simulink model "buck_simulation_1"  (R2023a)
settings: Solver=FixedStepAuto  StartTime=0.0  StopTime=0.5  FixedStep=1e-8  MaxStep=10e-9  RelTol=4e-3
libraries: spsSeriesRLCBranchLib x7, dspstat3 x6, spsDCVoltageSourceLib x2, spsMosfetLib x2, spsFourierLib x2, simulink x1, spsCurrentMeasurementLib x1, spsVoltageMeasurementLib x1, sps_lib x1
settings Model: Creator=13520  LastModifiedBy=13520

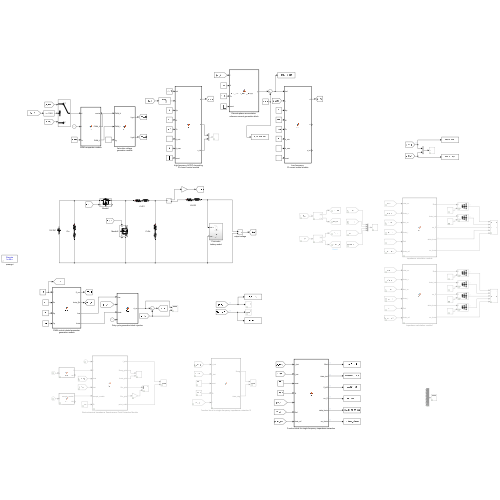
[thumbnail: Simulink's stored preview of the top-level diagram]
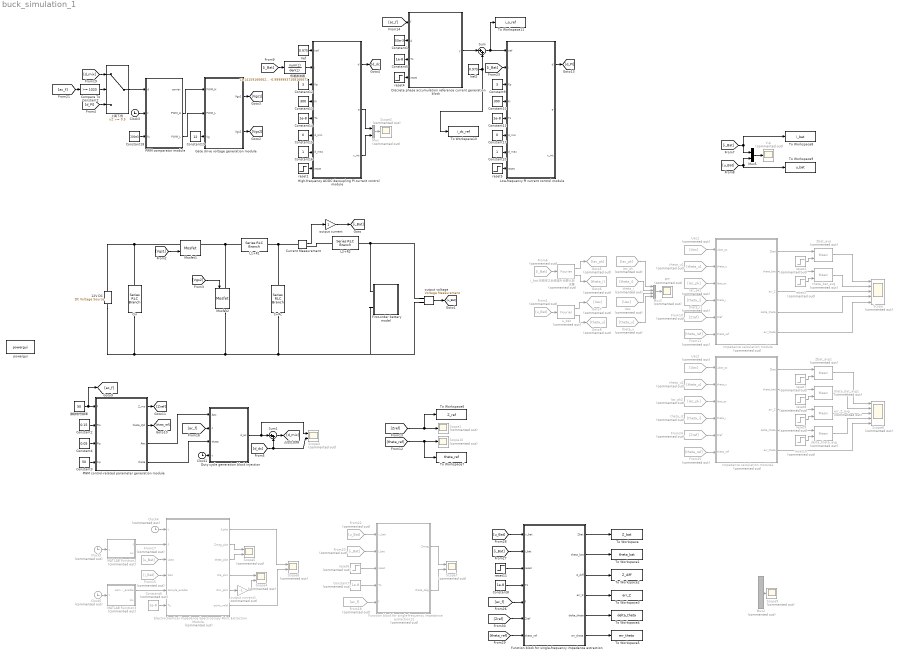
== system buck_simulation_1 ==
  12V DC : spsDCVoltageSourceLib/DC Voltage Source  Amplitude=12  Measurements=None
  C+Rc : spsSeriesRLCBranchLib/Series RLC Branch  LConnTagsString=__new0  RConnTagsString=__new0  BranchType=RC  Resistance=5e-1  Inductance=1e-3  SetiL0=off  InitialCurrent=0  Capacitance=220e-6  Setx0=off  InitialVoltage=0  Measurements=None
  Cin : spsSeriesRLCBranchLib/Series RLC Branch  LConnTagsString=__new0  RConnTagsString=__new0  BranchType=RC  Resistance=1  Inductance=1e-3  SetiL0=off  InitialCurrent=0  Capacitance=21e-6  Setx0=off  InitialVoltage=0  Measurements=None
  Clock1 : Clock
  Clock2 : Clock  Commented=on
  Clock3 : Clock
  Clock4 : Clock  Commented=on
  Clock5 : Clock  Commented=on
  Compare To Constant2 : simulink/Logic and Bit Operations/Compare To Constant  relop=>=  const=1020  OutDataTypeStr=boolean
  Constant1 : Constant  Value=50e-3
  Constant10 : Constant  Value=300
  Constant{5,8,11,14} (4 alike) : Constant  Value=1e-8
  Constant12 : Constant  Value=3
  Constant13 : Constant  Value=300
  Constant15 : Constant  Value=0
  Constant16 : Constant
  Constant17 : Constant  Value=0
  Constant18 : Constant  Value=200e3
  Constant19 : Constant  Value=12
  Constant2 : Constant  Value=0.15
  Constant20 : Constant
  Constant3 : Constant  Value=50
  Constant4 : Constant  Value=0.05
  Constant6 : Constant  Commented=on  Value=1e-8
  Constant7 : Constant  Commented=on  Value=1e-8
  Constant9 : Constant  Value=3
  Current Measurement : spsCurrentMeasurementLib/Current Measurement  PhasorSimulation=off  OutputType=Complex  PSBequivalent=0
  Discrete phase accumulation reference current generation block : MATLAB Function  TreatAsAtomicUnit=on
  Duty cycle generation block injection : MATLAB Function  TreatAsAtomicUnit=on
  Electrochemical Impedance Spectroscopy Point Extraction Module : MATLAB Function  Commented=on  TreatAsAtomicUnit=on
  FFT : Scope  Commented=on
  First-order battery model : Subsystem
  From1 : From  Commented=on  GotoTag=u_Bat
  From10 : From  Commented=on  GotoTag=Zref
  From11 : From  Commented=on  GotoTag=theta_ref
  From15 : From  Commented=on  GotoTag=i_Bat
  From17 : From  Commented=on  GotoTag=u_Bat
  From18 : From  Commented=on  GotoTag=ac_f
  From20 : From  Commented=on  GotoTag=i_Bat
  From22 : From  Commented=on  GotoTag=u_Bat
  From24 : From  Commented=on  GotoTag=Zref
  From25 : From  Commented=on  GotoTag=theta_ref
  From6 : From  Commented=on  GotoTag=i_Bat
  Function block for single-frequency impedance extraction : MATLAB Function  TreatAsAtomicUnit=on
  Function block for single-frequency impedance extraction12 : MATLAB Function  Commented=on  TreatAsAtomicUnit=on
  Gate drive voltage generation module : MATLAB Function  TreatAsAtomicUnit=on
  Goto5 : Goto  Commented=on  GotoTag=Iac_pk
  Goto6 : Goto  Commented=on  GotoTag=theta_i
  Goto7 : Goto  Commented=on  GotoTag=Uac
  Goto8 : Goto  Commented=on  GotoTag=theta_u
  High-frequency AC/DC decoupling PI current control module : MATLAB Function  TreatAsAtomicUnit=on  SystemSampleTime=1e-8
  Iac_pk : From  Commented=on  GotoTag=Iac_pk
  Iac_pk1 : From  Commented=on  GotoTag=Iac_pk
  Iac_pk2 : From  Commented=on  GotoTag=Iac_pk
  Impedance calculation module : MATLAB Function  Commented=on  TreatAsAtomicUnit=on
  Impedance calculation module1 : MATLAB Function  Commented=on  TreatAsAtomicUnit=on
  Iref : Constant  Value=0.975
  Iref2 : Constant  Value=0.975
  L1+R1 : spsSeriesRLCBranchLib/Series RLC Branch  LConnTagsString=__new0  RConnTagsString=__new0  BranchType=RL  Resistance=1e-1  Inductance=100e-6  SetiL0=off  InitialCurrent=0  Capacitance=1e-6  Setx0=off  InitialVoltage=0  Measurements=None
  L2+R2 : spsSeriesRLCBranchLib/Series RLC Branch  LConnTagsString=__new0  RConnTagsString=__new0  BranchType=RL  Resistance=16e-3  Inductance=15e-6  SetiL0=off  InitialCurrent=0  Capacitance=1e-6  Setx0=off  InitialVoltage=0  Measurements=None
  Low-frequency PI current control module : MATLAB Function  TreatAsAtomicUnit=on  SystemSampleTime=1e-8
  MATLAB Function2 : MATLAB Function  Commented=on  TreatAsAtomicUnit=on
  MATLAB Function3 : MATLAB Function  Commented=on  TreatAsAtomicUnit=on
  Mosfet1 : spsMosfetLib/Mosfet  Ron=0.1  Lon=0  Rd=0.01  Vfd=0  IC=0  Rs=1e5  Cs=inf  Measurements=on
  Mosfet2 : spsMosfetLib/Mosfet  Ron=0.1  Lon=0  Rd=0.01  Vfd=0  IC=0  Rs=1e5  Cs=inf  Measurements=on
  Mux : Mux  Commented=on  Inputs=2
  Mux1 : Mux  Commented=on
  Mux2 : Mux  Commented=on  Inputs=6
  Mux5 : Mux  Inputs=2
  PWM comparator module : MATLAB Function  TreatAsAtomicUnit=on
  PWM control-related parameter generation module : MATLAB Function  TreatAsAtomicUnit=on
  Scope : Scope  Commented=on  NumInputPorts=5
  Scope{1..2,9..10} (4 alike) : Scope  Commented=on
  Scope{3..7} (5 alike) : Scope  Commented=on  NumInputPorts=2
  Scope8 : Scope  Commented=on  NumInputPorts=5
  Sum : Sum  Inputs=|++
  Sum1 : Sum  Inputs=|++
  To Workspace : ToWorkspace  VariableName=Z_bat  SaveFormat=Timeseries  SampleTime=-1
  To Workspace1 : ToWorkspace  VariableName=theta_bat  SaveFormat=Timeseries  SampleTime=-1
  To Workspace10 : ToWorkspace  VariableName=i_dc_ref  SaveFormat=Timeseries  SampleTime=-1
  To Workspace11 : ToWorkspace  VariableName=i_o_ref  SaveFormat=Timeseries  SampleTime=-1
  To Workspace2 : ToWorkspace  VariableName=Z_diff  SaveFormat=Timeseries  SampleTime=-1
  To Workspace3 : ToWorkspace  VariableName=err_Z  SaveFormat=Timeseries  SampleTime=-1
  To Workspace4 : ToWorkspace  VariableName=delta_theta  SaveFormat=Timeseries  SampleTime=-1
  To Workspace5 : ToWorkspace  VariableName=err_theta  SaveFormat=Timeseries  SampleTime=-1
  To Workspace6 : ToWorkspace  VariableName=Z_ref  SaveFormat=Timeseries  SampleTime=-1
  To Workspace7 : ToWorkspace  VariableName=theta_ref  SaveFormat=Timeseries  SampleTime=-1
  To Workspace8 : ToWorkspace  VariableName=i_bat  SaveFormat=Timeseries  SampleTime=-1
  To Workspace9 : ToWorkspace  VariableName=u_bat  SaveFormat=Timeseries  SampleTime=-1
  Uac : From  Commented=on  GotoTag=Uac
  Uac1 : From  Commented=on  GotoTag=Uac
  Uac2 : From  Commented=on  GotoTag=Uac
  V-A : Scope  Commented=on
  Zbat_avg : dspstat3/Mean  Commented=on  run=on  reset_popup=Rising edge  directionMode=Each column  dimension=1  roiEnable=off  roiType=Rectangles  roiPortion=Entire ROI  roiOutput=Individual statistics for each ROI  roiFlag=off  roundingMode=Floor  overflowMode=off  outputDataTypeStr=Inherit: Same as accumulator  outputMin=[]  outputMax=[]  outputLastDataTypeStr=Inherit: Same as accumulator
  Zbat_avg1 : dspstat3/Mean  Commented=on  run=on  reset_popup=Rising edge  directionMode=Each column  dimension=1  roiEnable=off  roiType=Rectangles  roiPortion=Entire ROI  roiOutput=Individual statistics for each ROI  roiFlag=off  roundingMode=Floor  overflowMode=off  outputDataTypeStr=Inherit: Same as accumulator  outputMin=[]  outputMax=[]  outputLastDataTypeStr=Inherit: Same as accumulator
  delta_theta_avg : dspstat3/Mean  Commented=on  run=on  reset_popup=Rising edge  directionMode=Each column  dimension=1  roiEnable=off  roiType=Rectangles  roiPortion=Entire ROI  roiOutput=Individual statistics for each ROI  roiFlag=off  roundingMode=Floor  overflowMode=off  outputDataTypeStr=Inherit: Same as accumulator  outputMin=[]  outputMax=[]  outputLastDataTypeStr=Inherit: Same as accumulator
  err_Z_avg : dspstat3/Mean  Commented=on  run=on  reset_popup=Rising edge  directionMode=Each column  dimension=1  roiEnable=off  roiType=Rectangles  roiPortion=Entire ROI  roiOutput=Individual statistics for each ROI  roiFlag=off  roundingMode=Floor  overflowMode=off  outputDataTypeStr=Inherit: Same as accumulator  outputMin=[]  outputMax=[]  outputLastDataTypeStr=Inherit: Same as accumulator
  i_bat 改频率之后傅里叶也要从新设置 : spsFourierLib/Fourier  Commented=on  Freq=50  n=1  InInit=[0, 0]  Ts=1e-8
  output current : Gain
  output current1 : Gain  Commented=on  Gain=-1
  output voltage : spsVoltageMeasurementLib/Voltage Measurement  PhasorSimulation=off  OutputType=Complex  PSBequivalent=0
  powergui : sps_lib/powergui  Priority=1  SimulationMode=Discrete  SampleTime=1e-8  frequency=60  Iterations=50  frequencyindice=0  Pbase=100e6  ErrMax=1e-4  UnitsV=kV  UnitsW=MW  buscounter=0  FunctionMessages=off  echomessages=off  EnableUseOfTLC=off  CurrentSourceSwitches=off  DisableSnubberDevices=off  DisableRonSwitches=off  DisableVfSwitches=off  DisplayEquations=off  AutomaticDiscreteSolvers=off  SolverType=Tustin/Backward Euler (TBE)  Interpol=off  ExternalGateDelay=off  methode=off  Ts=100  x0status=blocks  SPID=on  SwTol=0  HookPort=off  NonlinearTolerance=1e-4  nMaxIteration=100  ContinueOnMaxIteration=off  RestoreLinks=warning  ResistiveCurrentMeasurement=off  Frange=[0:2:500]  Ylog=off  Xlog=on  ShowGrid=off  save=off  variable=ZData  structure=0  ZoomFFT=off  StartTime=0.0  cycles=1  DisplayStyle=1  fundamental=60  FreqAxis=off  MaxFrequency=1000  frequencyindicesteady=1  RmsSteady=1  display=off
  reset1 : Step  Time=0  Before=1  After=0  SampleTime=0
  reset{7..10} (4 alike) : Step  Commented=on  Time=0.05  SampleTime=1e-8
  reset11 : Step  Time=0.1  Before=1  After=0  SampleTime=0
  reset2 : Step  Commented=on  Time=0.25  SampleTime=1e-8
  reset3 : Step  Commented=on  Time=0.25  SampleTime=1e-8
  reset4 : Step  Time=0.05  Before=1  After=0  SampleTime=0
  reset5 : Step  Time=0  Before=1  After=0  SampleTime=0
  reset6 : Step  Commented=on  Time=0.1  Before=1  After=0  SampleTime=0
  theta_bat_avg : dspstat3/Mean  Commented=on  run=on  reset_popup=Rising edge  directionMode=Each column  dimension=1  roiEnable=off  roiType=Rectangles  roiPortion=Entire ROI  roiOutput=Individual statistics for each ROI  roiFlag=off  roundingMode=Floor  overflowMode=off  outputDataTypeStr=Inherit: Same as accumulator  outputMin=[]  outputMax=[]  outputLastDataTypeStr=Inherit: Same as accumulator
  theta_bat_avg1 : dspstat3/Mean  Commented=on  run=on  reset_popup=Rising edge  directionMode=Each column  dimension=1  roiEnable=off  roiType=Rectangles  roiPortion=Entire ROI  roiOutput=Individual statistics for each ROI  roiFlag=off  roundingMode=Floor  overflowMode=off  outputDataTypeStr=Inherit: Same as accumulator  outputMin=[]  outputMax=[]  outputLastDataTypeStr=Inherit: Same as accumulator
  theta_i : From  Commented=on  GotoTag=theta_i
  theta_i1 : From  Commented=on  GotoTag=theta_i
  theta_i2 : From  Commented=on  GotoTag=theta_i
  theta_u : From  Commented=on  GotoTag=theta_u
  theta_u1 : From  Commented=on  GotoTag=theta_u
  theta_u2 : From  Commented=on  GotoTag=theta_u
  u_bat : spsFourierLib/Fourier  Commented=on  Freq=50  n=1  InInit=[0, 0]  Ts=1e-8
  上高下低 : Switch  Threshold=0.5  SaturateOnIntegerOverflow=off  InputSameDT=off
  低通滤波器 : DiscreteTransferFcn  Numerator=[3.141591666629663e-07 3.141591666629663e-07]  Denominator=[1 -0.9999993716816667]  SampleTime=1e-8
  激励信号频率 : Constant  Value=50
  wires:
  Mux/1 -> Scope2/1
  [Vgs1] -> Mosfet1/1
  Constant12/1 -> High-frequency AC/DC decoupling PI current control module/3(Kp)
  Constant13/1 -> High-frequency AC/DC decoupling PI current control module/4(Ki)
  Constant14/1 -> High-frequency AC/DC decoupling PI current control module/5(Ts)
  Constant15/1 -> High-frequency AC/DC decoupling PI current control module/6(d_min)
  Constant16/1 -> High-frequency AC/DC decoupling PI current control module/7(d_max)
  reset1/1 -> High-frequency AC/DC decoupling PI current control module/8(reset)
  Constant19/1 -> Gate drive voltage generation module/3(Vg)
  PWM comparator module/2(PWM_H) -> Gate drive voltage generation module/1(PWM_H)
  PWM comparator module/3(PWM_L) -> Gate drive voltage generation module/2(PWM_L)
  Clock3/1 -> PWM comparator module/2(t)
  Constant18/1 -> PWM comparator module/3(fs)
  Gate drive voltage generation module/2(Vgs2) -> [Vgs2]
  Gate drive voltage generation module/1(Vgs1) -> [Vgs1]
  [Vgs2] -> Mosfet2/1
  Mux5/1 -> V-A/1
  output voltage/1 -> [u_Bat]
  Current Measurement/1 -> output current/1
  output current/1 -> [i_Bat]
  High-frequency AC/DC decoupling PI current control module/2(e) -> Mux/1
  High-frequency AC/DC decoupling PI current control module/3(x_int) -> Mux/2
  From1/1 -> u_bat/1
  From6/1 -> i_bat 改频率之后傅里叶也要从新设置/1
  [i_Bat] -> Mux5/1, To Workspace8/1
  [u_Bat] -> Mux5/2, To Workspace9/1
  i_bat 改频率之后傅里叶也要从新设置/1 -> Goto5/1
  i_bat 改频率之后傅里叶也要从新设置/2 -> Goto6/1
  u_bat/1 -> Goto7/1
  u_bat/2 -> Goto8/1
  Mux1/1 -> FFT/1
  Iac_pk/1 -> Mux1/1
  theta_i/1 -> Mux1/2
  Uac/1 -> Mux1/3
  theta_u/1 -> Mux1/4
  Uac1/1 -> Impedance calculation module/1(ubat_ac)
  Iac_pk1/1 -> Impedance calculation module/3(ibat_ac)
  theta_u1/1 -> Impedance calculation module/2(theta_u)
  theta_i1/1 -> Impedance calculation module/4(theta_i)
  From10/1 -> Impedance calculation module/5(Zref)
  Constant2/1 -> PWM control-related parameter generation module/2(Ro)
  Constant4/1 -> PWM control-related parameter generation module/3(Rp)
  Constant3/1 -> PWM control-related parameter generation module/4(Cp)
  PWM control-related parameter generation module/1(Z_mo) -> [Zref]
  From11/1 -> Impedance calculation module/6(theta_ref)
  PWM control-related parameter generation module/2(theta_Zjd) -> [theta_ref]
  [Zref] -> To Workspace6/1, Scope1/1
  [theta_ref] -> To Workspace7/1, Scope10/1
  reset2/1 -> Zbat_avg/2
  Impedance calculation module/1(Zbat) -> Zbat_avg/1
  reset3/1 -> theta_bat_avg/2
  Impedance calculation module/2(theta_bat) -> theta_bat_avg/1
  Zbat_avg/1 -> Scope/1
  theta_bat_avg/1 -> Scope/2
  Impedance calculation module/3(err_Z) -> Scope/3
  Impedance calculation module/4(delta_theta) -> Scope/4
  Impedance calculation module/5(err_theta) -> Scope/5
  [i_Bat] -> 低通滤波器/1
  Clock1/1 -> Duty cycle generation block injection/4(t)
  Iref/1 -> High-frequency AC/DC decoupling PI current control module/1(Iref)
  低通滤波器/1 -> High-frequency AC/DC decoupling PI current control module/2(i)
  PWM control-related parameter generation module/3(Aac) -> Duty cycle generation block injection/1(Aac)
  PWM control-related parameter generation module/4(theta) -> Duty cycle generation block injection/3(theta)
  [d_dc] -> Sum1/2, Scope3/2
  Sum1/1 -> [d_mix]
  Duty cycle generation block injection/1(d_ac) -> Scope3/1, Sum1/1
  High-frequency AC/DC decoupling PI current control module/1(d) -> [d_dc]
  Compare To Constant2/1 -> 上高下低/2
  上高下低/1 -> PWM comparator module/1(d)
  [ac_f] -> Compare To Constant2/1
  Constant11/1 -> Low-frequency PI current control module/5(Ts)
  Constant9/1 -> Low-frequency PI current control module/3(Kp)
  Constant17/1 -> Low-frequency PI current control module/6(d_min)
  Constant10/1 -> Low-frequency PI current control module/4(Ki)
  reset5/1 -> Low-frequency PI current control module/8(reset)
  Constant20/1 -> Low-frequency PI current control module/7(d_max)
  [ac_f] -> Duty cycle generation block injection/2(f)
  Low-frequency PI current control module/1(d) -> [d_PI]
  [d_mix] -> 上高下低/1
  [d_PI] -> 上高下低/3
  [i_Bat] -> Low-frequency PI current control module/2(i)
  Sum/1 -> To Workspace11/1, Low-frequency PI current control module/1(Iref)
  Iref2/1 -> Sum/2, To Workspace10/1
  Discrete phase accumulation reference current generation block/1(y) -> Sum/1
  [ac_f] -> Discrete phase accumulation reference current generation block/1(f)
  Constant1/1 -> Discrete phase accumulation reference current generation block/2(A)
  Constant5/1 -> Discrete phase accumulation reference current generation block/3(Ts)
  reset4/1 -> Discrete phase accumulation reference current generation block/4(reset)
  MATLAB Function3/1(sample_enable) -> Electrochemical Impedance Spectroscopy Point Extraction Module/5(sample_enable)
  Clock2/1 -> MATLAB Function2/1(t)
  Clock4/1 -> Electrochemical Impedance Spectroscopy Point Extraction Module/1(t)
  Clock5/1 -> MATLAB Function3/1(t)
  From17/1 -> Electrochemical Impedance Spectroscopy Point Extraction Module/3(ubat)
  From15/1 -> Electrochemical Impedance Spectroscopy Point Extraction Module/4(ibat)
  Constant6/1 -> Electrochemical Impedance Spectroscopy Point Extraction Module/6(Ts)
  Electrochemical Impedance Spectroscopy Point Extraction Module/4(Zre_plot) -> Scope4/1
  Electrochemical Impedance Spectroscopy Point Extraction Module/5(Zim_plot) -> output current1/1
  output current1/1 -> Scope4/2
  Electrochemical Impedance Spectroscopy Point Extraction Module/2(Zmag_plot) -> Scope5/1
  Electrochemical Impedance Spectroscopy Point Extraction Module/3(theta_plot) -> Scope5/2
  Electrochemical Impedance Spectroscopy Point Extraction Module/1(f_plot) -> Scope6/1
  Electrochemical Impedance Spectroscopy Point Extraction Module/6(point_valid) -> Scope6/2
  MATLAB Function2/1(f) -> Electrochemical Impedance Spectroscopy Point Extraction Module/2(f)
  激励信号频率/1 -> [ac_f], PWM control-related parameter generation module/1(f)
  From18/1 -> Function block for single-frequency impedance extraction12/5(f)
  Constant7/1 -> Function block for single-frequency impedance extraction12/4(Ts)
  From22/1 -> Function block for single-frequency impedance extraction12/1(v_bat)
  From20/1 -> Function block for single-frequency impedance extraction12/2(i_bat)
  reset6/1 -> Function block for single-frequency impedance extraction12/3(reset)
  Function block for single-frequency impedance extraction12/1(Zmag) -> Scope7/1
  Function block for single-frequency impedance extraction12/2(theta_deg) -> Scope7/2
  theta_bat_avg1/1 -> Scope8/2
  reset8/1 -> theta_bat_avg1/2
  Impedance calculation module1/2(theta_bat) -> theta_bat_avg1/1
  Impedance calculation module1/5(err_theta) -> Scope8/5
  Zbat_avg1/1 -> Scope8/1
  Impedance calculation module1/1(Zbat) -> Zbat_avg1/1
  Iac_pk2/1 -> Impedance calculation module1/3(ibat_ac)
  From24/1 -> Impedance calculation module1/5(Zref)
  From25/1 -> Impedance calculation module1/6(theta_ref)
  theta_u2/1 -> Impedance calculation module1/2(theta_u)
  theta_i2/1 -> Impedance calculation module1/4(theta_i)
  reset7/1 -> Zbat_avg1/2
  Uac2/1 -> Impedance calculation module1/1(ubat_ac)
  reset9/1 -> err_Z_avg/2
  Impedance calculation module1/3(err_Z) -> err_Z_avg/1
  err_Z_avg/1 -> Scope8/3
  reset10/1 -> delta_theta_avg/2
  Impedance calculation module1/4(delta_theta) -> delta_theta_avg/1
  delta_theta_avg/1 -> Scope8/4
  Constant8/1 -> Function block for single-frequency impedance extraction/4(Ts)
  reset11/1 -> Function block for single-frequency impedance extraction/3(reset)
  [u_Bat] -> Function block for single-frequency impedance extraction/1(v_bat)
  [i_Bat] -> Function block for single-frequency impedance extraction/2(i_bat)
  [ac_f] -> Function block for single-frequency impedance extraction/5(f)
  Mux2/1 -> Scope9/1
  Function block for single-frequency impedance extraction/4(err_Z) -> To Workspace3/1
  Function block for single-frequency impedance extraction/2(theta_bat) -> To Workspace1/1
  Function block for single-frequency impedance extraction/1(Zbat) -> To Workspace/1
  Function block for single-frequency impedance extraction/5(delta_theta) -> To Workspace4/1
  Function block for single-frequency impedance extraction/6(err_theta) -> To Workspace5/1
  [Zref] -> Function block for single-frequency impedance extraction/6(Zref)
  [theta_ref] -> Function block for single-frequency impedance extraction/7(theta_ref)
  Function block for single-frequency impedance extraction/3(Z_diff) -> To Workspace2/1
  connections:
  12V DC/RConn1 -- Mosfet1/LConn1 -- Cin/LConn1
  L1+R1/LConn1 -- Mosfet2/LConn1 -- Mosfet1/RConn1
  C+Rc/LConn1 -- Current Measurement/LConn1 -- L1+R1/RConn1
  12V DC/LConn1 -- Cin/RConn1 -- Mosfet2/RConn1 -- output voltage/LConn2 -- First-order battery model/LConn2 -- C+Rc/RConn1
  L2+R2/LConn1 -- Current Measurement/RConn1
  output voltage/LConn1 -- First-order battery model/LConn1 -- L2+R2/RConn1

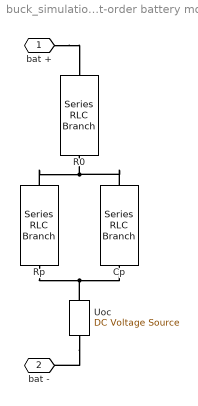
== system buck_simulation_1/First-order battery model ==
  Cp : spsSeriesRLCBranchLib/Series RLC Branch  LConnTagsString=__new0  RConnTagsString=__new0  BranchType=C  Resistance=0.5  Inductance=1e-3  SetiL0=off  InitialCurrent=0  Capacitance=50  Setx0=off  InitialVoltage=0  Measurements=None
  R0 : spsSeriesRLCBranchLib/Series RLC Branch  LConnTagsString=__new0  RConnTagsString=__new0  BranchType=R  Resistance=15e-2  Inductance=1e-3  SetiL0=off  InitialCurrent=0  Capacitance=1e-6  Setx0=off  InitialVoltage=0  Measurements=None
  Rp : spsSeriesRLCBranchLib/Series RLC Branch  LConnTagsString=__new0  RConnTagsString=__new0  BranchType=R  Resistance=5e-2  Inductance=1e-3  SetiL0=off  InitialCurrent=0  Capacitance=1e-6  Setx0=off  InitialVoltage=0  Measurements=None
  Uoc : spsDCVoltageSourceLib/DC Voltage Source  Amplitude=3.6  Measurements=None
  bat + : PMIOPort  Side=Left
  bat - : PMIOPort  Port=2  Side=Left
  connections:
  Rp/RConn1 -- Uoc/RConn1 -- Cp/RConn1
  Rp/LConn1 -- Cp/LConn1 -- R0/RConn1
  bat +/RConn1 -- R0/LConn1
  Uoc/LConn1 -- bat -/RConn1

== matlab function buck_simulation_1/High-frequency AC//DC decoupling PI current control module ==
  settings: updateMethod=DISCRETE
  data: Iref input; d output; i input; Kp input; Ki input; Ts input; d_min input; d_max input; reset input; e output; x_int output
function [d, e, x_int] = fcn(Iref, i, Kp, Ki, Ts, d_min, d_max, reset)
% High-frequency AC/DC decoupling PI current control module
% Inputs:
%   Iref  - Reference current
%   i     - Actual current
%   Kp    - Proportional coefficient
%   Ki    - Integral coefficient
%   Ts    - Sampling period
%   d_min - Lower duty cycle limit
%   d_max - Upper duty cycle limit
%   reset - Reset signal
%
% Outputs:
%   d     - Duty cycle output
%   e     - Current error
%   x_int - Integral state

persistent int_e

if isempty(int_e)
    int_e = 0;
end

if reset > 0.5
    int_e = 0;
end

% Current error
e = Iref - i;

% Integral term
int_e = int_e + e * Ts;

% PI output
d = Kp * e + Ki * int_e;

% Duty cycle saturation
if d > d_max
    d = d_max;
elseif d < d_min
    d = d_min;
end

% Output integral state
x_int = int_e;
end

== matlab function buck_simulation_1/Gate drive voltage generation module ==
  data: PWM_H input; Vgs1 output; PWM_L input; Vg input; Vgs2 output
function [Vgs1, Vgs2] = fcn(PWM_H, PWM_L, Vg)
% Gate drive voltage generation module
% Inputs:
%   PWM_H - High-side PWM (recommended input: 0 or 1)
%   PWM_L - Low-side PWM (recommended input: 0 or 1)
%   Vg    - Gate-source drive voltage amplitude, for example 12 V
%
% Outputs:
%   Vgs1  - Gate-source drive voltage of S1
%   Vgs2  - Gate-source drive voltage of S2

% Limit the high-side PWM to 0~1
if PWM_H >= 0.5
    h = 1;
else
    h = 0;
end

% Limit the low-side PWM to 0~1
if PWM_L >= 0.5
    l = 1;
else
    l = 0;
end

% Drive amplitude protection
if Vg < 0
    Vg_use = 0;
else
    Vg_use = Vg;
end

% Output gate-source voltage
Vgs1 = h * Vg_use;
Vgs2 = l * Vg_use;
end

== matlab function buck_simulation_1/MATLAB Function2 ==
  data: t input; f output; sw output
function [f, sw] = fcn(t)
% 扫频块 / 交流激励电流频率生成模块
% 输入:
%   t  - 当前仿真时间
%
% 输出:
%   f  - 当前扫频频率
%   sw - 附录1原始控制标志

% 附录1中的频率数组
fx = [1 25000 20000 10000 5000 2000 1000 500 50 10];

% 附录1中的时间切换点数组
tx = [0 0.1 0.69 1.09 1.64 2.29 3.24 4.69 6.09 8];

% 附录1中的控制标志数组
swx = [0 1 1 1 1 1 1 1 1 1];

% 默认输出最后一个频点
f = fx(10);
sw = swx(10);

for i = 1:length(tx)-1
    if t >= tx(i) && t <= tx(i+1)
        f = fx(i);
        sw = swx(i);
        break;
    end
end
end

== matlab function buck_simulation_1/MATLAB Function3 ==
  data: t input; sample_enable output; idx output
function [sample_enable, idx] = fcn(t)
% 扫频采样窗口生成模块
% 输入:
%   t - 当前仿真时间
%
% 输出:
%   sample_enable - 当前频点是否允许采样
%   idx           - 当前频点索引

% 附录1时间切换点
tx = [0 0.1 0.69 1.09 1.64 2.29 3.24 4.69 6.09 8];

sample_enable = 0;
idx = 0;

for i = 1:length(tx)-1
    if t >= tx(i) && t < tx(i+1)
        idx = i;
        t1 = tx(i);
        t2 = tx(i+1);

        % 只在该频点区间后20%允许采样
        if t >= t1 + 0.8*(t2 - t1)
            sample_enable = 1;
        end
        break;
    end
end
end

== matlab function buck_simulation_1/Function block for single-frequency impedance extraction12 ==
  data: v_bat input; Zmag output; i_bat input; reset input; Ts input; f input; theta_deg output
function [Zmag, theta_deg] = fcn(v_bat, i_bat, reset, Ts, f)
% 用于单频阻抗提的取函数块
% 输入:
%   v_bat   - 电池端电压
%   i_bat   - 电池端电流
%   reset   - 复位信号，1=清零并等待，0=开始测量
%   Ts      - 离散步长
%   f       - 当前激励频率(Hz)
%
% 输出:
%   Zmag      - 当前频点阻抗模
%   theta_deg - 当前频点阻抗角(度)
%
% 说明:
%   1) 该模块采用单频同步检波法，不需要额外 Fourier 块
%   2) reset=1 时清空内部状态，适合在 PI 稳定阶段保持复位
%   3) reset 拉低后，模块开始对当前频率进行多周期累计
%   4) 达到设定测量周期数后，输出并保持该频点结果

% ========= 可调参数 =========
N_cycle_measure = 3;    % 测量周期数，可改为 2~5
I_min = 1e-9;           % 防止除零
% ===========================

persistent phi
persistent t_acc
persistent vsum_sin vsum_cos isum_sin isum_cos
persistent sample_count
persistent Zmag_hold theta_hold

if isempty(phi)
    phi = 0;
    t_acc = 0;
    vsum_sin = 0;
    vsum_cos = 0;
    isum_sin = 0;
    isum_cos = 0;
    sample_count = 0;
    Zmag_hold = 0;
    theta_hold = 0;
end

% 默认输出保持上一次有效值
Zmag = Zmag_hold;
theta_deg = theta_hold;

% 频率非法时直接返回
if f <= 0 || Ts <= 0
    Zmag = 0;
    theta_deg = 0;
    return;
end

% 复位：清空累计器，但不输出测量结果
if reset > 0.5
    phi = 0;
    t_acc = 0;
    vsum_sin = 0;
    vsum_cos = 0;
    isum_sin = 0;
    isum_cos = 0;
    sample_count = 0;
    Zmag_hold = 0;
    theta_hold = 0;

    Zmag = 0;
    theta_deg = 0;
    return;
end

% 当前角频率
w = 2*pi*f;

% 相位累加
phi = phi + w*Ts;

% 相位限制到 0~2pi
if phi >= 2*pi
    phi = phi - 2*pi*floor(phi/(2*pi));
end

% 参考正弦/余弦
ref_sin = sin(phi);
ref_cos = cos(phi);

% 同步检波累计
vsum_sin = vsum_sin + v_bat * ref_sin;
vsum_cos = vsum_cos + v_bat * ref_cos;

isum_sin = isum_sin + i_bat * ref_sin;
isum_cos = isum_cos + i_bat * ref_cos;

sample_count = sample_count + 1;
t_acc = t_acc + Ts;

% 达到设定测量时长后计算一次结果
T_measure = N_cycle_measure / f;

if t_acc >= T_measure
    % 提取当前频率分量
    Vsin = 2 * vsum_sin / sample_count;
    Vcos = 2 * vsum_cos / sample_count;

    Isin = 2 * isum_sin / sample_count;
    Icos = 2 * isum_cos / sample_count;

    % 幅值
    Vamp = sqrt(Vsin*Vsin + Vcos*Vcos);
    Iamp = sqrt(Isin*Isin + Icos*Icos);

    % 相位
    theta_v = atan2(Vcos, Vsin);
    theta_i = atan2(Icos, Isin);

    % 阻抗计算
    if Iamp > I_min
        Zmag_hold = Vamp / Iamp;
        theta_hold = (theta_v - theta_i) * 180 / pi;
    else
        Zmag_hold = 0;
        theta_hold = 0;
    end

    % 相角限制到 -180 ~ 180 deg
    while theta_hold > 180
        theta_hold = theta_hold - 360;
    end
    while theta_hold < -180
        theta_hold = theta_hold + 360;
    end

    % 输出最新结果
    Zmag = Zmag_hold;
    theta_deg = theta_hold;

    % 计算完成后，重新开始累计下一轮
    % 如果你只想每次 reset 后测一次并保持，也可以把下面这段删掉
    phi = 0;
    t_acc = 0;
    vsum_sin = 0;
    vsum_cos = 0;
    isum_sin = 0;
    isum_cos = 0;
    sample_count = 0;
end
end

== matlab function buck_simulation_1/Impedance calculation module1 ==
  data: ubat_ac input; Zbat output; theta_u input; ibat_ac input; theta_i input; Zref input; theta_ref input; theta_bat output; err_Z output; delta_theta output; err_theta output
function [Zbat, theta_bat, err_Z, delta_theta, err_theta] = fcn(ubat_ac, theta_u, ibat_ac, theta_i, Zref, theta_ref)
% 阻抗计算模块（抑制 100 Hz 误差振荡优化版）
% 输入:
%   ubat_ac   - 锂电池两端交流响应电压幅值
%   theta_u   - 锂电池两端交流响应电压相位（度）
%   ibat_ac   - 锂电池输入交流电流幅值
%   theta_i   - 锂电池输入交流电流相位（度）
%   Zref      - 标准阻抗模
%   theta_ref - 标准阻抗角（度）
%
% 输出:
%   Zbat        - 实测阻抗模（平滑后）
%   theta_bat   - 实测阻抗角（平滑后，度）
%   err_Z       - 阻抗模误差百分比（平滑后）
%   delta_theta - 阻抗角绝对误差（平滑后，度）
%   err_theta   - 阻抗角误差百分比（平滑后）

% =========================
% 可调参数
% =========================
eps_I = 1e-12;          % 防止电流幅值过小
eps_Z = 1e-12;          % 防止参考阻抗过小
theta_ref_min = 1e-3;   % 参考相角过小时，不计算百分比误差

alpha_Z = 0.02;         % 阻抗模平滑系数，越小越稳，建议 0.01~0.05
alpha_th = 0.02;        % 阻抗角平滑系数，越小越稳，建议 0.01~0.05
beta_err = 0.02;        % 误差平滑系数，越小越稳，建议 0.01~0.05

% =========================
% 持久变量
% =========================
persistent is_init
persistent Z_filt
persistent th_cos_filt th_sin_filt
persistent eZ_filt eTh_filt

if isempty(is_init)
    is_init = 0;
    Z_filt = 0;
    th_cos_filt = 1;   % 对应 0 度
    th_sin_filt = 0;
    eZ_filt = 0;
    eTh_filt = 0;
end

% =========================
% 默认输出
% =========================
Zbat = Z_filt;
theta_bat = atan2d(th_sin_filt, th_cos_filt);
err_Z = 0;
delta_theta = abs(eTh_filt);
err_theta = 0;

% =========================
% 输入合法性检查
% =========================
if ~isfinite(ubat_ac) || ~isfinite(theta_u) || ...
   ~isfinite(ibat_ac) || ~isfinite(theta_i) || ...
   ~isfinite(Zref) || ~isfinite(theta_ref) || ...
   abs(ibat_ac) < eps_I

    % 输入异常时直接保持上一时刻结果
    Zbat = Z_filt;
    theta_bat = atan2d(th_sin_filt, th_cos_filt);

    if abs(Zref) > eps_Z
        err_Z = abs(eZ_filt) / abs(Zref) * 100;
    else
        err_Z = 0;
    end

    delta_theta = abs(eTh_filt);

    if abs(theta_ref) > theta_ref_min
        err_theta = abs(eTh_filt) / abs(theta_ref) * 100;
    else
        err_theta = 0;
    end
    return;
end

% =========================
% 1) 用相量法计算瞬时阻抗
% =========================
Uac = abs(ubat_ac);
Iac = abs(ibat_ac);

u_re = Uac * cosd(theta_u);
u_im = Uac * sind(theta_u);

i_re = Iac * cosd(theta_i);
i_im = Iac * sind(theta_i);

den = i_re*i_re + i_im*i_im;

if den < eps_I^2
    % 电流过小，保持上一结果
    Zbat = Z_filt;
    theta_bat = atan2d(th_sin_filt, th_cos_filt);

    if abs(Zref) > eps_Z
        err_Z = abs(eZ_filt) / abs(Zref) * 100;
    else
        err_Z = 0;
    end

    delta_theta = abs(eTh_filt);

    if abs(theta_ref) > theta_ref_min
        err_theta = abs(eTh_filt) / abs(theta_ref) * 100;
    else
        err_theta = 0;
    end
    return;
end

% 复数除法 Z = U / I
z_re = (u_re*i_re + u_im*i_im) / den;
z_im = (u_im*i_re - u_re*i_im) / den;

Z_inst = sqrt(z_re*z_re + z_im*z_im);
theta_inst = atan2d(z_im, z_re);

% 规范到 [-180, 180]
while theta_inst > 180
    theta_inst = theta_inst - 360;
end
while theta_inst < -180
    theta_inst = theta_inst + 360;
end

% =========================
% 2) 首次有效输入时直接初始化
% =========================
if is_init == 0
    Z_filt = Z_inst;
    th_cos_filt = cosd(theta_inst);
    th_sin_filt = sind(theta_inst);

    % 初始带符号误差
    eZ_filt = Z_inst - abs(Zref);

    eTh_tmp = theta_inst - theta_ref;
    while eTh_tmp > 180
        eTh_tmp = eTh_tmp - 360;
    end
    while eTh_tmp < -180
        eTh_tmp = eTh_tmp + 360;
    end
    eTh_filt = eTh_tmp;

    is_init = 1;
end

% =========================
% 3) 对阻抗模和平滑相角做滤波
%    相角不能直接平滑角度值，应用 cos/sin 平滑避免跳边界
% =========================
Z_filt = (1 - alpha_Z) * Z_filt + alpha_Z * Z_inst;

th_cos_inst = cosd(theta_inst);
th_sin_inst = sind(theta_inst);

th_cos_filt = (1 - alpha_th) * th_cos_filt + alpha_th * th_cos_inst;
th_sin_filt = (1 - alpha_th) * th_sin_filt + alpha_th * th_sin_inst;

theta_filt = atan2d(th_sin_filt, th_cos_filt);

while theta_filt > 180
    theta_filt = theta_filt - 360;
end
while theta_filt < -180
    theta_filt = theta_filt + 360;
end

% =========================
% 4) 误差先按“带符号”形式平滑，再取绝对值输出
%    这样不会把 50 Hz 纹波直接整流成 100 Hz
% =========================
Zref_use = abs(Zref);
eZ_inst = Z_filt - Zref_use;
eZ_filt = (1 - beta_err) * eZ_filt + beta_err * eZ_inst;

eTh_inst = theta_filt - theta_ref;
while eTh_inst > 180
    eTh_inst = eTh_inst - 360;
end
while eTh_inst < -180
    eTh_inst = eTh_inst + 360;
end

eTh_filt = (1 - beta_err) * eTh_filt + beta_err * eTh_inst;

% =========================
% 5) 输出
% =========================
Zbat = Z_filt;
theta_bat = theta_filt;

if Zref_use > eps_Z
    err_Z = abs(eZ_filt) / Zref_use * 100;
else
    err_Z = 0;
end

delta_theta = abs(eTh_filt);

if abs(theta_ref) > theta_ref_min
    err_theta = abs(eTh_filt) / abs(theta_ref) * 100;
else
    err_theta = 0;
end

end

== matlab function buck_simulation_1/Impedance calculation module ==
  data: ubat_ac input; Zbat output; theta_u input; ibat_ac input; theta_i input; Zref input; theta_ref input; theta_bat output; err_Z output; delta_theta output; err_theta output
function [Zbat, theta_bat, err_Z, delta_theta, err_theta] = fcn(ubat_ac, theta_u, ibat_ac, theta_i, Zref, theta_ref)
% 阻抗计算模块（单频单点版）
% 输入:
%   ubat_ac   - 锂电池两端交流响应电压幅值
%   theta_u   - 锂电池两端交流响应电压相位（度）
%   ibat_ac   - 锂电池输入交流电流幅值
%   theta_i   - 锂电池输入交流电流相位（度）
%   Zref      - 标准阻抗模
%   theta_ref - 标准阻抗角（度）
%
% 输出:
%   Zbat        - 实测阻抗模
%   theta_bat   - 实测阻抗角（度）
%   err_Z       - 阻抗模误差百分比
%   delta_theta - 阻抗角绝对误差（度）
%   err_theta   - 阻抗角误差百分比

% 防止分母为 0
eps_val = 1e-12;

% 1) 实测阻抗模
if abs(ibat_ac) < eps_val
    Zbat = 0;
else
    Zbat = ubat_ac / ibat_ac;
end

% 2) 实测阻抗角
theta_bat = theta_u - theta_i;

% 3) 阻抗模误差百分比
if abs(Zref) < eps_val
    err_Z = 0;
else
    err_Z = abs(Zbat - Zref) / abs(Zref) * 100;
end

% 4) 阻抗角绝对误差
delta_theta = abs(theta_bat - theta_ref);

% 5) 阻抗角误差百分比
if abs(theta_ref) < eps_val
    err_theta = 0;
else
    err_theta = delta_theta / abs(theta_ref) * 100;
end
end

== matlab function buck_simulation_1/Function block for single-frequency impedance extraction ==
  data: v_bat input; Zbat output; i_bat input; reset input; Ts input; f input; theta_bat output; Z_diff output; err_Z output; delta_theta output; err_theta output; Zref input; theta_ref input
function [Zbat, theta_bat,Z_diff, err_Z, delta_theta, err_theta ] = fcn(v_bat, i_bat, reset, Ts, f, Zref, theta_ref)
% Function block for single-frequency impedance extraction (reference error calculation + Z_diff output)
% Inputs:
%   v_bat     - Battery terminal voltage (original time-domain signal, including DC + AC)
%   i_bat     - Battery terminal current (original time-domain signal, including DC + AC)
%   reset     - Reset signal, 1 = clear and wait, 0 = start measurement
%   Ts        - Discrete time step
%   f         - Current excitation frequency (Hz)
%   Zref      - Reference impedance magnitude
%   theta_ref - Reference impedance angle (degrees)
%
% Outputs:
%   Zbat        - Measured impedance magnitude
%   theta_bat   - Measured impedance angle (degrees)
%   err_Z       - Percentage error of impedance magnitude
%   delta_theta - Absolute error of impedance angle (degrees)
%   err_theta   - Percentage error of impedance angle
%   Z_diff      - Impedance magnitude difference Zbat - Zref
%
% Notes:
%   1) Use single-frequency synchronous detection to extract directly from the original v_bat and i_bat
%   2) Clear and wait when reset = 1
%   3) After reset is pulled low, discard several cycles first, then measure over integer cycles
%   4) After one measurement, latch and hold the result until the next reset or frequency change
%   5) Calculate the errors in real time according to the input Zref and theta_ref

% =========================
% Adjustable parameters
% =========================
N_cycle_ignore  = 1;      % Number of cycles discarded before measurement starts
N_cycle_measure = 6;      % Number of cycles actually used for measurement
Iamp_min        = 1e-8;   % Minimum AC current threshold to prevent division by zero
eps_val         = 1e-12;  % Small-value threshold

% =========================
% Persistent variables
% =========================
persistent phi
persistent cycle_count
persistent meas_done
persistent f_last

persistent sum_v sum_i
persistent sum_vs sum_vc
persistent sum_is sum_ic
persistent sum_s sum_c
persistent N

persistent Z_hold theta_hold
persistent errZ_hold dtheta_hold errtheta_hold
persistent Zdiff_hold

if isempty(phi)
    phi = 0;
    cycle_count = 0;
    meas_done = 0;
    f_last = 0;

    sum_v  = 0;
    sum_i  = 0;
    sum_vs = 0;
    sum_vc = 0;
    sum_is = 0;
    sum_ic = 0;
    sum_s  = 0;
    sum_c  = 0;
    N = 0;

    Z_hold = 0;
    theta_hold = 0;
    errZ_hold = 0;
    dtheta_hold = 0;
    errtheta_hold = 0;
    Zdiff_hold = 0;
end

% Default output keeps the last valid value
Zbat        = Z_hold;
theta_bat   = theta_hold;
err_Z       = errZ_hold;
delta_theta = dtheta_hold;
err_theta   = errtheta_hold;
Z_diff      = Zdiff_hold;

% Invalid input protection
if (Ts <= 0) || (f <= 0)
    Zbat        = 0;
    theta_bat   = 0;
    err_Z       = 0;
    delta_theta = 0;
    err_theta   = 0;
    Z_diff      = 0;
    return;
end

% When reset is active: clear all states and wait
if reset > 0.5
    phi = 0;
    cycle_count = 0;
    meas_done = 0;
    f_last = f;

    sum_v  = 0;
    sum_i  = 0;
    sum_vs = 0;
    sum_vc = 0;
    sum_is = 0;
    sum_ic = 0;
    sum_s  = 0;
    sum_c  = 0;
    N = 0;

    Z_hold = 0;
    theta_hold = 0;
    errZ_hold = 0;
    dtheta_hold = 0;
    errtheta_hold = 0;
    Zdiff_hold = 0;

    Zbat        = 0;
    theta_bat   = 0;
    err_Z       = 0;
    delta_theta = 0;
    err_theta   = 0;
    Z_diff      = 0;
    return;
end

% If the frequency changes, restart the measurement for this frequency point
if abs(f - f_last) > max(eps_val, 1e-9 * max(1, abs(f_last)))
    phi = 0;
    cycle_count = 0;
    meas_done = 0;
    f_last = f;

    sum_v  = 0;
    sum_i  = 0;
    sum_vs = 0;
    sum_vc = 0;
    sum_is = 0;
    sum_ic = 0;
    sum_s  = 0;
    sum_c  = 0;
    N = 0;

    Z_hold = 0;
    theta_hold = 0;
    errZ_hold = 0;
    dtheta_hold = 0;
    errtheta_hold = 0;
    Zdiff_hold = 0;

    Zbat        = 0;
    theta_bat   = 0;
    err_Z       = 0;
    delta_theta = 0;
    err_theta   = 0;
    Z_diff      = 0;
end

% If the measurement has been completed, directly hold the output
if meas_done > 0.5
    Zbat        = Z_hold;
    theta_bat   = theta_hold;
    err_Z       = errZ_hold;
    delta_theta = dtheta_hold;
    err_theta   = errtheta_hold;
    Z_diff      = Zdiff_hold;
    return;
end

% =========================
% Single-frequency synchronous detection
% Read the reference first, then advance the phase
% =========================
ref_sin = sin(phi);
ref_cos = cos(phi);

% Start accumulation only after the ignored cycles have ended
if cycle_count >= N_cycle_ignore
    sum_v  = sum_v  + v_bat;
    sum_i  = sum_i  + i_bat;

    sum_vs = sum_vs + v_bat * ref_sin;
    sum_vc = sum_vc + v_bat * ref_cos;

    sum_is = sum_is + i_bat * ref_sin;
    sum_ic = sum_ic + i_bat * ref_cos;

    sum_s  = sum_s  + ref_sin;
    sum_c  = sum_c  + ref_cos;

    N = N + 1;
end

% Advance the phase
phi = phi + 2*pi*f*Ts;

% Count using complete cycles
while phi >= 2*pi
    phi = phi - 2*pi;
    cycle_count = cycle_count + 1;
end

% =========================
% After reaching the specified measurement cycles, calculate once and latch
% =========================
if (cycle_count >= (N_cycle_ignore + N_cycle_measure)) && (N > 0)

    % ---- Explicitly remove DC leakage ----
    mean_v = sum_v / N;
    mean_i = sum_i / N;

    Vsin = 2 * (sum_vs - mean_v * sum_s) / N;
    Vcos = 2 * (sum_vc - mean_v * sum_c) / N;

    Isin = 2 * (sum_is - mean_i * sum_s) / N;
    Icos = 2 * (sum_ic - mean_i * sum_c) / N;

    % ---- Amplitude ----
    Vamp = sqrt(Vsin*Vsin + Vcos*Vcos);
    Iamp = sqrt(Isin*Isin + Icos*Icos);

    % ---- Phase ----
    theta_v = atan2(Vcos, Vsin);
    theta_i = atan2(Icos, Isin);

    % ---- Impedance ----
    if Iamp > Iamp_min
        Z_hold = Vamp / Iamp;
        theta_hold = (theta_v - theta_i) * 180 / pi;
    else
        Z_hold = 0;
        theta_hold = 0;
    end

    % Limit the phase angle to [-180, 180]
    while theta_hold > 180
        theta_hold = theta_hold - 360;
    end
    while theta_hold < -180
        theta_hold = theta_hold + 360;
    end

    % ---- Impedance magnitude difference ----
    Zdiff_hold = Z_hold - Zref;

    % =========================
    % Error calculation
    % =========================

    % Percentage error of impedance magnitude
    if abs(Zref) > eps_val
        errZ_hold = abs(Z_hold - Zref) / abs(Zref) * 100;
    else
        errZ_hold = 0;
    end

    % Absolute phase angle error (considering angle wrapping)
    angle_diff = theta_hold - theta_ref;
    while angle_diff > 180
        angle_diff = angle_diff - 360;
    end
    while angle_diff < -180
        angle_diff = angle_diff + 360;
    end
    dtheta_hold = abs(angle_diff);

    % Percentage error of phase angle
    if abs(theta_ref) > eps_val
        errtheta_hold = dtheta_hold / abs(theta_ref) * 100;
    else
        errtheta_hold = 0;
    end

    % Latch completed
    meas_done = 1;
end

% Output latched values
Zbat        = Z_hold;
theta_bat   = theta_hold;
err_Z       = errZ_hold;
delta_theta = dtheta_hold;
err_theta   = errtheta_hold;
Z_diff      = Zdiff_hold;

end

== matlab function buck_simulation_1/PWM comparator module ==
  data: d input; carrier output; t input; fs input; PWM_H output; PWM_L output
function [carrier, PWM_H, PWM_L] = fcn(d, t, fs)
% PWM comparator module
% Inputs:
%   d       - Duty cycle input, expected range 0~1
%   t       - Current simulation time
%   fs      - Switching frequency
%
% Outputs:
%   carrier - Normalized sawtooth carrier, range 0~1
%   PWM_H   - High-side PWM output (0 or 1)
%   PWM_L   - Low-side PWM output (0 or 1)

% Prevent abnormal inputs
if d > 1
    d_use = 1;
elseif d < 0
    d_use = 0;
else
    d_use = d;
end

% Prevent invalid frequency
if fs <= 0
    carrier = 0;
    PWM_H = 0;
    PWM_L = 1;
    return;
end

% PWM period
T_pwm = 1 / fs;

% Normalized sawtooth carrier: linearly rises from 0 to nearly 1 in each period
carrier = mod(t, T_pwm) / T_pwm;

% Compare to obtain the high-side PWM
if d_use >= carrier
    PWM_H = 1;
else
    PWM_H = 0;
end

% Ideal complementary low-side PWM
PWM_L = 1 - PWM_H;
end

== matlab function buck_simulation_1/Duty cycle generation block injection ==
  data: Aac input; d_ac output; f input; theta input; t input
function d_ac = fcn(Aac, f, theta, t)
% Duty cycle injection generation block
% Inputs:
%   Aac   - Amplitude of the AC duty cycle component
%   f     - AC excitation frequency
%   theta - Phase of the AC duty cycle component (radians)
%   t     - Current system time
%
% Outputs:
%   d_ac  - AC duty cycle signal

d_ac = Aac * sin(2*pi*f*t + theta);
end

== matlab function buck_simulation_1/Discrete phase accumulation reference current generation block ==
  data: f input; y output; A input; Ts input; reset input
function y = LF_Current_Sine_PhaseAcc(f, A, Ts, reset)
% Discrete phase accumulation reference current generation block
% Inputs:
%   f     - Current frequency (Hz)
%   A     - Sine amplitude (A)
%   Ts    - Sampling period (s)
%   reset - Reset signal (phase is cleared when >0.5)
%
% Outputs:
%   y     - Low-frequency AC reference current

persistent theta

% Initialization
if isempty(theta)
    theta = 0;
end

% Input protection
if f < 0
    f_use = 0;
else
    f_use = f;
end

if A < 0
    A_use = 0;
else
    A_use = A;
end

if Ts <= 0
    y = 0;
    return;
end

% Reset: clear the phase and restart from the zero point
if reset > 0.5
    theta = 0;
    y = 0;
    return;
end

% Output the sine value corresponding to the current phase
y = A_use * sin(theta);

% Phase recursion
theta = theta + 2*pi*f_use*Ts;

% Constrain the phase to [-pi, pi] to prevent numerical growth
if theta > pi
    theta = theta - 2*pi;
elseif theta < -pi
    theta = theta + 2*pi;
end
end

== matlab function buck_simulation_1/Low-frequency PI current control module ==
  settings: updateMethod=DISCRETE
  data: Iref input; d output; i input; Kp input; Ki input; Ts input; d_min input; d_max input; reset input; e output; x_int output
function [d, e, x_int] = fcn(Iref, i, Kp, Ki, Ts, d_min, d_max, reset)
% Low-frequency PI current control module
% Inputs:
%   Iref  - Reference current
%   i     - Actual current
%   Kp    - Proportional coefficient
%   Ki    - Integral coefficient
%   Ts    - Sampling period
%   d_min - Lower duty cycle limit
%   d_max - Upper duty cycle limit
%   reset - Reset signal
%
% Outputs:
%   d     - Duty cycle output
%   e     - Current error
%   x_int - Integral state

persistent int_e

if isempty(int_e)
    int_e = 0;
end

if reset > 0.5
    int_e = 0;
end

% Current error
e = Iref - i;

% Integral term
int_e = int_e + e * Ts;

% PI output
d = Kp * e + Ki * int_e;

% Duty cycle saturation
if d > d_max
    d = d_max;
elseif d < d_min
    d = d_min;
end

% Output integral state
x_int = int_e;
end

== matlab function buck_simulation_1/PWM control-related parameter generation module ==
  data: f input; Z_mo output; theta_Zjd output; Aac output; theta output; Ro input; Rp input; Cp input
function [Z_mo, theta_Zjd, Aac, theta] = fcn(f, Ro, Rp, Cp)
% PWM control-related parameter generation module
% Inputs:
%   f           - AC excitation current frequency
%   Ro          - Ohmic internal resistance of the first-order equivalent circuit
%   Rp          - Polarization resistance of the first-order equivalent circuit
%   Cp          - Polarization capacitance of the first-order equivalent circuit
%
% Outputs:
%   Z_mo        - Impedance magnitude of the first-order equivalent circuit
%   theta_Zjd   - Impedance angle of the first-order equivalent circuit (degrees)
%   Aac         - Duty cycle signal amplitude
%   theta       - Duty cycle signal phase (radians)

w = 2*pi*f;

% Impedance calculation of the first-order equivalent circuit
X_c = 1/(w*Cp*1i);
Z = Ro + (Rp*X_c)/(Rp + X_c);   % Impedance of the first-order equivalent circuit

Z_mo = abs(Z);                  % Impedance magnitude of the first-order equivalent circuit
theta_Zrad = angle(Z);          % Impedance angle of the first-order equivalent circuit (radians)
theta_Zjd = theta_Zrad*180/pi;  % Impedance angle of the first-order equivalent circuit (degrees)

% The following formulas are used for the target duty cycle function under high-frequency conditions
L1 = 100e-6;    % Inductor 1
R1 = 0.102;
L2 = 15e-6;     % Inductor 2
R2 = 0.0178;
C  = 220e-6;    % Output capacitor
Rc = 0.5;
Iac = 0.05;    % Amplitude of the AC disturbance reference current
Ui = 12;        % Input voltage

m1 = (w*(L1+L2)*Iac)/(Ui);
m2 = w*w*L1*C*((w*L2*Iac - w*Rc*R2*C*Iac)/((1 + w*w*C*C*Rc*Rc)*Ui));
m3 = w*R1*C*((w*w*Rc*L2*C*Iac + R2*Iac)/((1 + w*w*Rc*Rc*C*C)*Ui));
m = m1 - m2 + m3;

n1 = (R1+R2)*Iac/Ui;
n2 = w*w*L1*C*((w*w*Rc*L2*C*Iac + R2*Iac)/((1 + w*w*C*C*Rc*Rc)*Ui));
n3 = w*R1*C*((w*L2*Iac - w*Rc*R2*C*Iac)/((1 + w*w*C*C*Rc*Rc)*Ui));
n = n1 - n2 - n3;

Aac = sqrt(m^2 + n^2);

if n < 0
    theta = atan(m/n) + pi;
else
    theta = atan(m/n);
end

== matlab function buck_simulation_1/Electrochemical Impedance Spectroscopy Point Extraction Module ==
  data: t input; f_plot output; f input; ubat input; ibat input; sample_enable input; Ts input; Zmag_plot output; theta_plot output; Zre_plot output; Zim_plot output; point_valid output
function [f_plot, Zmag_plot, theta_plot, Zre_plot, Zim_plot, point_valid] = fcn(t, f, ubat, ibat, sample_enable, Ts)
% 电化学阻抗谱点提取模块（基于原始时域电压电流）
% 输入:
%   t             - 当前仿真时间
%   f             - 当前频率
%   ubat          - 电池原始端电压时域信号
%   ibat          - 电池原始输入电流时域信号
%   sample_enable - 当前频点是否允许采样
%   Ts            - 仿真步长
%
% 输出:
%   f_plot        - 记录下来的频率点
%   Zmag_plot     - 记录下来的阻抗模
%   theta_plot    - 记录下来的阻抗角（度）
%   Zre_plot      - 记录下来的阻抗实部
%   Zim_plot      - 记录下来的阻抗虚部
%   point_valid   - 当前时刻是否刚刚输出了一个新谱点

persistent last_en
persistent sum_u_sin sum_u_cos sum_i_sin sum_i_cos N
persistent f_hold Zmag_hold theta_hold Zre_hold Zim_hold

eps_val = 1e-12;

if isempty(last_en)
    last_en = 0;

    sum_u_sin = 0;
    sum_u_cos = 0;
    sum_i_sin = 0;
    sum_i_cos = 0;
    N = 0;

    f_hold = 0;
    Zmag_hold = 0;
    theta_hold = 0;
    Zre_hold = 0;
    Zim_hold = 0;
end

point_valid = 0;

% 参考正弦/余弦
w = 2*pi*f;
s_ref = sin(w*t);
c_ref = cos(w*t);

% 1) 采样窗口刚打开：清零累积器
if (sample_enable > 0.5) && (last_en <= 0.5)
    sum_u_sin = 0;
    sum_u_cos = 0;
    sum_i_sin = 0;
    sum_i_cos = 0;
    N = 0;
end

% 2) 采样窗口内：持续累积
if sample_enable > 0.5
    sum_u_sin = sum_u_sin + ubat * s_ref;
    sum_u_cos = sum_u_cos + ubat * c_ref;

    sum_i_sin = sum_i_sin + ibat * s_ref;
    sum_i_cos = sum_i_cos + ibat * c_ref;

    N = N + 1;
end

% 3) 采样窗口刚关闭：统一计算并输出一个谱点
if (sample_enable <= 0.5) && (last_en > 0.5) && (N > 0)
    u_s = sum_u_sin / N;
    u_c = sum_u_cos / N;

    i_s = sum_i_sin / N;
    i_c = sum_i_cos / N;

    % 同步提取得到当前频点电压/电流幅值
    Uac = 2 * sqrt(u_s*u_s + u_c*u_c);
    Iac = 2 * sqrt(i_s*i_s + i_c*i_c);

    % 相位（先弧度，后转角度）
    theta_u_rad = atan2(u_c, u_s);
    theta_i_rad = atan2(i_c, i_s);

    theta_u_deg = theta_u_rad * 180 / pi;
    theta_i_deg = theta_i_rad * 180 / pi;

    % 频点阻抗
    if Iac < eps_val
        Zmag = 0;
    else
        Zmag = Uac / Iac;
    end

    theta_deg = theta_u_deg - theta_i_deg;

    % 规范到 [-180, 180]
    while theta_deg > 180
        theta_deg = theta_deg - 360;
    end
    while theta_deg < -180
        theta_deg = theta_deg + 360;
    end

    % 锁存输出
    f_hold = f;
    Zmag_hold = Zmag;
    theta_hold = theta_deg;
    Zre_hold = Zmag_hold * cosd(theta_hold);
    Zim_hold = Zmag_hold * sind(theta_hold);

    point_valid = 1;
end

last_en = sample_enable;

% 保持输出直到下一个频点更新
f_plot = f_hold;
Zmag_plot = Zmag_hold;
theta_plot = theta_hold;
Zre_plot = Zre_hold;
Zim_plot = Zim_hold;
end
